simulink model "setMotorsPID"  (R2019a)
settings: Solver=FixedStepAuto  StartTime=0.0  StopTime=10.0  RelTol=1e-3  EnableMultiTasking=on
undefined symbols (not defined in the file or in its folder): DiscIntNeverNeededParam
libraries: simulink x2
settings Model: Creator=florian  LastModifiedBy=florian
settings SolverCC: PositivePriorityOrder=on
settings OptimizationCC: EnhancedBackFolding=on  PassReuseOutputArgsAs=Individual arguments  MaxStackSize=64  OptimizeBlockOrder=speed  DifferentSizesBufferReuse=on  OptimizationCustomize=off
settings DebuggingCC: ParameterTunabilityLossMsg=error
settings HardwareCC: ProdBitPerPointer=32  ProdBitPerSizeT=32  ProdBitPerPtrDiffT=32  ProdLargestAtomicInteger=Long  ProdLargestAtomicFloat=Double  ProdWordSize=32  ProdLongLongMode=on  ProdHWDeviceType=ARM Compatible->ARM Cortex
settings SFSimCC: MATLABDynamicMemAlloc=off
settings RTWCC: SystemTargetFile=ert.tlc  HardwareBoard=Raspberry Pi  TLCOptions="-aInlineSetEventsForThisBaseRateFcn=TLC_FALSE -aSuppressMultiTaskScheduler=TLC_FALSE  -aRateBasedStepFcn=0"  TemplateMakefile=ert_default_tmf  GenerateReport=on  Toolchain=GNU GCC Raspberry Pi  BuildConfiguration=Faster Runs  IncludeHyperlinkInReport=on  LaunchReport=on  GenerateTraceInfo=on  GenerateTraceReport=on  GenerateTraceReportSl=on  GenerateTraceReportSf=on  GenerateTraceReportEml=on
settings CodeAppCC: ForceParamTrailComments=on  IgnoreCustomStorageClasses=off  OperatorAnnotations=on  SimulinkDataObjDesc=on  SFDataObjDesc=on  InsertBlockDesc=on
settings ERTTargetCC: SupportVariableSizeSignals=on

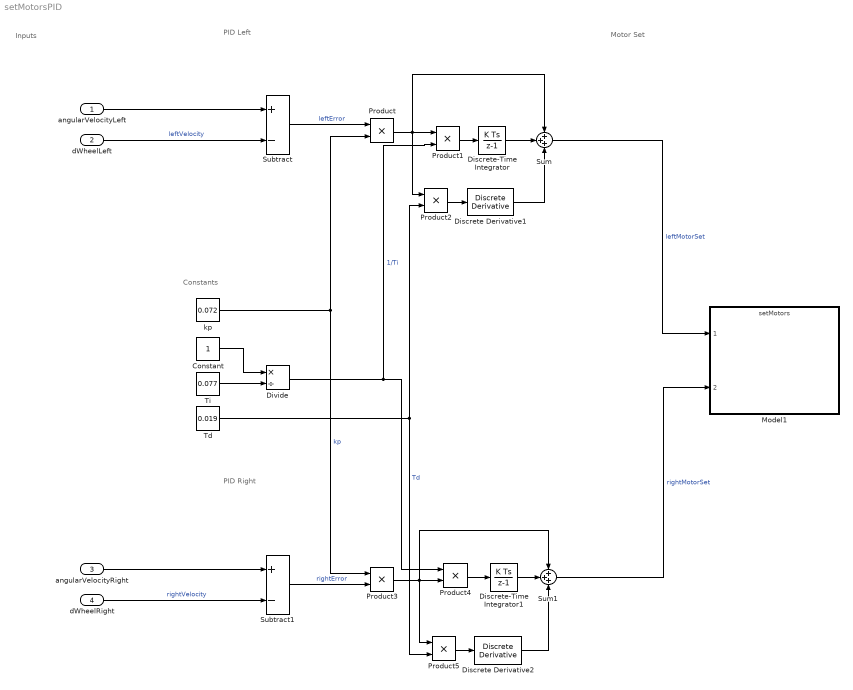
== system setMotorsPID ==
  note: Motor Set
  note: Inputs
  note: Constants
  note: PID Left
  note: PID Right
  angularVelocityLeft : Inport
  dWheelLeft : Inport  Port=2
  angularVelocityRight : Inport  Port=3
  dWheelRight : Inport  Port=4
  Constant : Constant
  Discrete Derivative1 : simulink/Discrete/Discrete Derivative  gainval=1  ICPrevScaledInput=0.0  OutMin=[]  OutMax=[]  OutDataType=fixdt(1, 16)  OutScaling=2^-10  DoSatur=off
  Discrete Derivative2 : simulink/Discrete/Discrete Derivative  gainval=1  ICPrevScaledInput=0.0  OutMin=[]  OutMax=[]  OutDataType=fixdt(1, 16)  OutScaling=2^-10  DoSatur=off
  Discrete-Time Integrator : DiscreteIntegrator  gainval=1  SampleTime=-1  ICPrevOutput=DiscIntNeverNeededParam  ICPrevScaledInput=DiscIntNeverNeededParam
  Discrete-Time Integrator1 : DiscreteIntegrator  gainval=1  SampleTime=-1  ICPrevOutput=DiscIntNeverNeededParam  ICPrevScaledInput=DiscIntNeverNeededParam
  Divide : Product  Inputs=*/
  Model1 : ModelReference  ModelNameDialog=setMotors.slx  SimulationMode=Normal  ModelReferenceVersion=1.7
  Product{,1..5} (6 alike) : Product
  Subtract : Sum  Inputs=+-
  Subtract1 : Sum  Inputs=+-
  Sum : Sum  Inputs=+++
  Sum1 : Sum  Inputs=+++
  Td : Constant  Value=0.019
  Ti : Constant  Value=0.077
  kp : Constant  Value=0.072
  wires:
  angularVelocityLeft/1 -> Subtract/1
  dWheelLeft/1 -> Subtract/2  "leftVelocity"
  Subtract/1 -> Product/1  "leftError"
  Product/1 -> Product2/1, Product1/1, Sum/1
  Discrete-Time Integrator/1 -> Sum/2
  Product1/1 -> Discrete-Time Integrator/1
  Discrete Derivative1/1 -> Sum/3
  Product2/1 -> Discrete Derivative1/1
  Sum/1 -> Model1/1  "leftMotorSet"
  Td/1 -> Product5/2, Product2/2  "Td"
  kp/1 -> Product3/1, Product/2  "kp"
  Discrete-Time Integrator1/1 -> Sum1/2
  Sum1/1 -> Model1/2  "rightMotorSet"
  Discrete Derivative2/1 -> Sum1/3
  Product5/1 -> Discrete Derivative2/1
  angularVelocityRight/1 -> Subtract1/1
  Subtract1/1 -> Product3/2  "rightError"
  Product3/1 -> Product4/2, Sum1/1, Product5/1
  dWheelRight/1 -> Subtract1/2  "rightVelocity"
  Product4/1 -> Discrete-Time Integrator1/1
  Ti/1 -> Divide/2
  Constant/1 -> Divide/1
  Divide/1 -> Product4/1, Product1/2  "1/Ti"
